simulink model "Controlador_PID_de_movimiento_discreto"  (R2023b)
settings: Solver=VariableStepAuto  StartTime=0.0  StopTime=14  RelTol=1e-3
values from neighbouring files (symbols this model uses):
  alpha_Cu = 3.9e-3    (= 0.0039)    [definicio_cte.m]
  b_a = 0.0396    [definicio_cte.m]
  b_eq = b_m + b_l/(r^2)    (= 1.98611111111e-05)    [definicio_cte.m]
  C_ts = 0.818    [definicio_cte.m]
  g = 9.80665    [definicio_cte.m]
  J_eq = J_m + J_l/(r^2)    (= 1.97847222222e-05)    [definicio_cte.m]
  k_l = m*l_cm + m_l*l_l    (= 0.25)    [definicio_cte.m]
  K_omega_2 = 3.0720e7    (= 30720000)    [definicio_cte.m]
  K_sa = 31.656    [definicio_cte.m]
  K_theta_2 = 9600    [definicio_cte.m]
  K_theta_i = 3.2768e10    (= 32768000000)    [definicio_cte.m]
  L_d = 6.6e-3    (= 0.0066)    [definicio_cte.m]
  L_ls = 0.8e-3    (= 0.0008)    [definicio_cte.m]
  L_q = 5.8e-3    (= 0.0058)    [definicio_cte.m]
  lambda_m = 0.016    [definicio_cte.m]
  lim_inf = -sqrt(2) * 48 / sqrt(3)    [definicio_cte.m]
  lim_sup = sqrt(2) * 48 / sqrt(3)    [definicio_cte.m]
  P_p = 3    [definicio_cte.m]
  r = 120    [definicio_cte.m]
  R_0 = 5000 * L_ls    (= 4)    [definicio_cte.m]
  R_d = 5000 * L_d    (= 33)    [definicio_cte.m]
  R_q = 5000 * L_q    (= 29)    [definicio_cte.m]
  R_sREF = 1.02    [definicio_cte.m]
  R_tsamb = 146.7    [definicio_cte.m]
  T_amb = 25    [definicio_cte.m]
  T_sREF = 20    [definicio_cte.m]
  tau = 20    [definicio_cte.m]
  Ts = 1.256e-4    (= 0.0001256)    [definicio_cte.m]
  w_modul = 6000*4    (= 24000)    [definicio_cte.m]
  wn_i = 6000*3    (= 18000)    [definicio_cte.m]
  wn_theta = 2000*3    (= 6000)    [definicio_cte.m]
  xita_i = 1    [definicio_cte.m]
  xita_modul = 1    [definicio_cte.m]
  xita_theta = 1    [definicio_cte.m]
undefined symbols (not defined in the file or in its folder): K_sia, magnitude
libraries: simulink x16
(part 2 of 2)

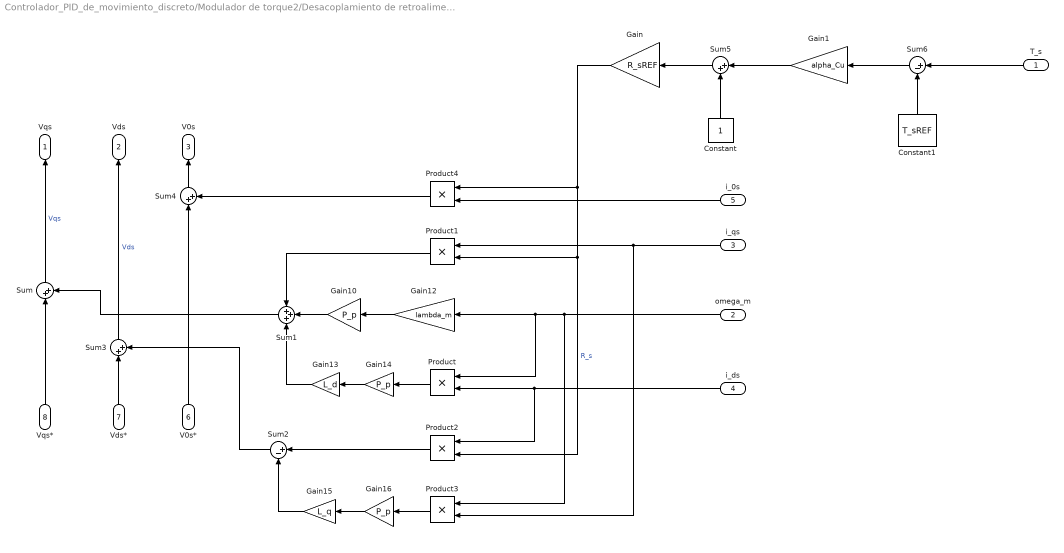
== system Controlador_PID_de_movimiento_discreto/Modulador de torque2/Desacoplamiento de retroalimentaciones fisicas naturales ==
  T_s : Inport
  omega_m : Inport  Port=2
  i_qs : Inport  Port=3
  i_ds : Inport  Port=4
  i_0s : Inport  Port=5
  V0s* : Inport  Port=6
  Vds* : Inport  Port=7
  Vqs* : Inport  Port=8
  Constant : Constant
  Constant1 : Constant  Value=T_sREF
  Gain : Gain  Gain=R_sREF
  Gain1 : Gain  Gain=alpha_Cu
  Gain10 : Gain  Gain=P_p
  Gain12 : Gain  Gain=lambda_m
  Gain13 : Gain  Gain=L_d
  Gain14 : Gain  Gain=P_p
  Gain15 : Gain  Gain=L_q
  Gain16 : Gain  Gain=P_p
  Product{,1..4} (5 alike) : Product
  Sum{,3..5} (4 alike) : Sum  Inputs=|++
  Sum1 : Sum  Inputs=+++
  Sum2 : Sum  Inputs=|+-
  Sum6 : Sum  Inputs=|+-
  Vqs : Outport
  Vds : Outport  Port=2
  V0s : Outport  Port=3
  wires:
  Gain10/1 -> Sum1/2
  Gain13/1 -> Sum1/3
  Gain12/1 -> Gain10/1
  i_qs/1 -> Product3/2, Product1/1
  i_ds/1 -> Product2/1, Product/2
  Gain16/1 -> Gain15/1
  Product2/1 -> Sum2/1
  Product3/1 -> Gain16/1
  Gain/1 -> Product2/2, Product1/2, Product4/1  "R_s"
  Gain15/1 -> Sum2/2
  Product1/1 -> Sum1/1
  Sum2/1 -> Sum3/2
  Sum1/1 -> Sum/2
  Product/1 -> Gain14/1
  omega_m/1 -> Product3/1, Product/1, Gain12/1
  Gain14/1 -> Gain13/1
  Sum3/1 -> Vds/1  "Vds"
  Sum/1 -> Vqs/1  "Vqs"
  i_0s/1 -> Product4/2
  Product4/1 -> Sum4/2
  Sum4/1 -> V0s/1
  Constant1/1 -> Sum6/2
  T_s/1 -> Sum6/1
  Constant/1 -> Sum5/2
  Sum5/1 -> Gain/1
  Sum6/1 -> Gain1/1
  Gain1/1 -> Sum5/1
  Vqs*/1 -> Sum/1
  Vds*/1 -> Sum3/1
  V0s*/1 -> Sum4/1

== system Controlador_PID_de_movimiento_discreto/Modulador de torque2/Lazo de corriente ==
  i_qs : Inport
  i_ds : Inport  Port=2
  i_0s : Inport  Port=3
  iqs* : Inport  Port=4
  ids* : Inport  Port=5
  i0s* : Inport  Port=6
  Gain10 : Gain  Gain=R_d
  Gain12 : Gain  Gain=R_0
  Gain9 : Gain  Gain=R_q
  Sum : Sum  Inputs=|-+
  Sum1 : Sum  Inputs=|-+
  Sum2 : Sum  Inputs=|-+
  V0s* : Outport
  Vds* : Outport  Port=2
  Vqs* : Outport  Port=3
  wires:
  Gain9/1 -> Vqs*/1  "Vqs*"
  Sum/1 -> Gain9/1
  Gain10/1 -> Vds*/1  "Vds*"
  i_qs/1 -> Sum/1
  ids*/1 -> Sum1/2
  i_0s/1 -> Sum2/1
  Sum2/1 -> Gain12/1
  Sum1/1 -> Gain10/1
  i0s*/1 -> Sum2/2
  iqs*/1 -> Sum/2
  i_ds/1 -> Sum1/1
  Gain12/1 -> V0s*/1  "V0s*"

== system Controlador_PID_de_movimiento_discreto/Modulador de torque2/Lazo de torque ==
  omega_m : Inport
  T_m'* : Inport  Port=2
  g : Inport  Port=3
  i_ds : Inport  Port=4
  theta_m : Inport  Port=5
  Constant4 : Constant  Value=L_d
  Constant5 : Constant  Value=L_q
  Constant6 : Constant  Value=lambda_m
  Divide1 : Product  Inputs=*/
  Gain16 : Gain  Gain=b_eq
  Gain17 : Gain  Gain=1/r
  Gain18 : Gain  Gain=k_l
  Gain19 : Gain  Gain=1/r
  Gain20 : Gain  Gain=P_p
  Gain21 : Gain  Gain=3/2
  Product1 : Product
  Product3 : Product
  Sin1 : Trigonometry
  Sum3 : Sum  Inputs=+++
  Sum4 : Sum  Inputs=-+
  Sum5 : Sum  Inputs=|++
  iqs* : Outport
  wires:
  theta_m/1 -> Gain17/1
  Product1/1 -> Sum3/3
  Constant6/1 -> Sum5/2
  Gain16/1 -> Sum3/2
  T_m'*/1 -> Sum3/1
  Gain21/1 -> Divide1/2
  g/1 -> Product1/2
  Constant5/1 -> Sum4/1
  Product3/1 -> Sum5/1
  Sum5/1 -> Gain20/1
  Gain18/1 -> Gain19/1
  Sum3/1 -> Divide1/1
  Divide1/1 -> iqs*/1  "iqs*"
  Gain20/1 -> Gain21/1
  Sum4/1 -> Product3/2
  Gain19/1 -> Product1/1
  Gain17/1 -> Sin1/1
  omega_m/1 -> Gain16/1
  Sin1/1 -> Gain18/1
  i_ds/1 -> Product3/1
  Constant4/1 -> Sum4/2

== system Controlador_PID_de_movimiento_discreto/Subsystem10/Subsystem ==
  u_a : Inport
  Gain10 : Gain  Gain=w_modul
  Gain12 : Gain  Gain=xita_modul
  Gain13 : Gain  Gain=2
  Gain14 : Gain  Gain=(w_modul)^2
  Gain9 : Gain  Gain=(w_modul)^2
  Integrator : Integrator
  Integrator1 : Integrator
  Sum : Sum  Inputs=+--
  y_a : Outport
  wires:
  Integrator1/1 -> y_a/1, Gain14/1  "x_1 = y"
  Integrator/1 -> Gain10/1, Integrator1/1  "x_2 = x_1'"
  Gain12/1 -> Gain13/1
  Gain13/1 -> Sum/3
  Sum/1 -> Integrator/1  "y' = x_2'"
  Gain9/1 -> Sum/1
  Gain10/1 -> Gain12/1
  Gain14/1 -> Sum/2
  u_a/1 -> Gain9/1

== system Controlador_PID_de_movimiento_discreto/Subsystem3/Subsystem ==
  u_a : Inport
  Gain10 : Gain  Gain=w_modul
  Gain12 : Gain  Gain=xita_modul
  Gain13 : Gain  Gain=2
  Gain14 : Gain  Gain=(w_modul)^2
  Gain9 : Gain  Gain=(w_modul)^2
  Integrator : Integrator
  Integrator1 : Integrator
  Sum : Sum  Inputs=+--
  y_a : Outport
  wires:
  Integrator1/1 -> y_a/1, Gain14/1  "x_1 = y"
  Integrator/1 -> Gain10/1, Integrator1/1  "x_2 = x_1'"
  Gain12/1 -> Gain13/1
  Gain13/1 -> Sum/3
  Sum/1 -> Integrator/1  "y' = x_2'"
  Gain9/1 -> Sum/1
  Gain10/1 -> Gain12/1
  Gain14/1 -> Sum/2
  u_a/1 -> Gain9/1

== system Controlador_PID_de_movimiento_discreto/Subsystem4/Subsystem ==
  u_a : Inport
  Gain10 : Gain  Gain=w_modul
  Gain12 : Gain  Gain=xita_modul
  Gain13 : Gain  Gain=2
  Gain14 : Gain  Gain=(w_modul)^2
  Gain9 : Gain  Gain=(w_modul)^2
  Integrator : Integrator
  Integrator1 : Integrator
  Sum : Sum  Inputs=+--
  y_a : Outport
  wires:
  u_a/1 -> Gain9/1
  Gain14/1 -> Sum/2
  Gain10/1 -> Gain12/1
  Gain9/1 -> Sum/1
  Sum/1 -> Integrator/1  "y' = x_2'"
  Gain13/1 -> Sum/3
  Gain12/1 -> Gain13/1
  Integrator/1 -> Integrator1/1, Gain10/1  "x_2 = x_1'"
  Integrator1/1 -> Gain14/1, y_a/1  "x_1 = y"

== system Controlador_PID_de_movimiento_discreto/Subsystem5/Subsystem ==
  u_a : Inport
  Gain10 : Gain  Gain=w_modul
  Gain12 : Gain  Gain=xita_modul
  Gain13 : Gain  Gain=2
  Gain14 : Gain  Gain=(w_modul)^2
  Gain9 : Gain  Gain=(w_modul)^2
  Integrator : Integrator
  Integrator1 : Integrator
  Sum : Sum  Inputs=+--
  y_a : Outport
  wires:
  Integrator1/1 -> y_a/1, Gain14/1  "x_1 = y"
  Integrator/1 -> Gain10/1, Integrator1/1  "x_2 = x_1'"
  Gain12/1 -> Gain13/1
  Gain13/1 -> Sum/3
  Sum/1 -> Integrator/1  "y' = x_2'"
  Gain9/1 -> Sum/1
  Gain10/1 -> Gain12/1
  Gain14/1 -> Sum/2
  u_a/1 -> Gain9/1

== system Controlador_PID_de_movimiento_discreto/Subsystem8/Subsystem ==
  u_a : Inport
  Gain10 : Gain  Gain=w_modul
  Gain12 : Gain  Gain=xita_modul
  Gain13 : Gain  Gain=2
  Gain14 : Gain  Gain=(w_modul)^2
  Gain9 : Gain  Gain=(w_modul)^2
  Integrator : Integrator
  Integrator1 : Integrator
  Sum : Sum  Inputs=+--
  y_a : Outport
  wires:
  Integrator1/1 -> y_a/1, Gain14/1  "x_1 = y"
  Integrator/1 -> Gain10/1, Integrator1/1  "x_2 = x_1'"
  Gain12/1 -> Gain13/1
  Gain13/1 -> Sum/3
  Sum/1 -> Integrator/1  "y' = x_2'"
  Gain9/1 -> Sum/1
  Gain10/1 -> Gain12/1
  Gain14/1 -> Sum/2
  u_a/1 -> Gain9/1

== system Controlador_PID_de_movimiento_discreto/Subsystem9/Subsystem ==
  u_a : Inport
  Gain10 : Gain  Gain=w_modul
  Gain12 : Gain  Gain=xita_modul
  Gain13 : Gain  Gain=2
  Gain14 : Gain  Gain=(w_modul)^2
  Gain9 : Gain  Gain=(w_modul)^2
  Integrator : Integrator
  Integrator1 : Integrator
  Sum : Sum  Inputs=+--
  y_a : Outport
  wires:
  u_a/1 -> Gain9/1
  Gain14/1 -> Sum/2
  Gain10/1 -> Gain12/1
  Gain9/1 -> Sum/1
  Sum/1 -> Integrator/1  "y' = x_2'"
  Gain13/1 -> Sum/3
  Gain12/1 -> Gain13/1
  Integrator/1 -> Integrator1/1, Gain10/1  "x_2 = x_1'"
  Integrator1/1 -> Gain14/1, y_a/1  "x_1 = y"

== system Controlador_PID_de_movimiento_discreto/observador de estados 1/Integrador discreto ==
  u : Inport
  Gain : Gain  Gain=Ts/2
  Sum : Sum  Inputs=|++
  Sum1 : Sum  Inputs=|++
  Unit Delay : UnitDelay  SampleTime=Ts  HasFrameUpgradeWarning=on
  Unit Delay1 : UnitDelay  SampleTime=Ts  HasFrameUpgradeWarning=on
  y : Outport
  wires:
  Unit Delay/1 -> Sum1/2
  Gain/1 -> Sum1/1
  Unit Delay1/1 -> Sum/2
  u/1 -> Unit Delay1/1, Sum/1
  Sum1/1 -> y/1, Unit Delay/1
  Sum/1 -> Gain/1

== system Controlador_PID_de_movimiento_discreto/observador de estados 1/Integrador discreto1 ==
  u : Inport
  Gain : Gain  Gain=Ts/2
  Sum : Sum  Inputs=|++
  Sum1 : Sum  Inputs=|++
  Unit Delay : UnitDelay  SampleTime=Ts  HasFrameUpgradeWarning=on
  Unit Delay1 : UnitDelay  SampleTime=Ts  HasFrameUpgradeWarning=on
  y : Outport
  wires:
  Sum/1 -> Gain/1
  Sum1/1 -> Unit Delay/1, y/1
  u/1 -> Sum/1, Unit Delay1/1
  Unit Delay1/1 -> Sum/2
  Gain/1 -> Sum1/1
  Unit Delay/1 -> Sum1/2

== system Controlador_PID_de_movimiento_discreto/observador de estados 1/Integrador discreto2 ==
  u : Inport
  Gain : Gain  Gain=Ts/2
  Sum : Sum  Inputs=|++
  Sum1 : Sum  Inputs=|++
  Unit Delay : UnitDelay  SampleTime=Ts  HasFrameUpgradeWarning=on
  Unit Delay1 : UnitDelay  SampleTime=Ts  HasFrameUpgradeWarning=on
  y : Outport
  wires:
  Unit Delay/1 -> Sum1/2
  Gain/1 -> Sum1/1
  Unit Delay1/1 -> Sum/2
  u/1 -> Unit Delay1/1, Sum/1
  Sum1/1 -> y/1, Unit Delay/1
  Sum/1 -> Gain/1

== system Controlador_PID_de_movimiento_discreto/./Subsistema Electromagnético/corriente_i_0s ==
  v_0s : Inport
  R_s : Inport  Port=2
  Gain : Gain  Gain=1/L_ls
  Integrator : Integrator
  Product : Product
  Sum : Sum  Inputs=+-
  i_0s : Outport
  wires:
  Sum/1 -> Gain/1
  Gain/1 -> Integrator/1  "i'_0s"
  Integrator/1 -> i_0s/1, Product/2
  Product/1 -> Sum/2
  v_0s/1 -> Sum/1
  R_s/1 -> Product/1

== system Controlador_PID_de_movimiento_discreto/./Subsistema Electromagnético/corriente_i_ds ==
  v_ds : Inport
  i_qs : Inport  Port=2
  omega_m : Inport  Port=3
  R_s : Inport  Port=4
  Gain : Gain  Gain=L_q
  Gain1 : Gain  Gain=P_p
  Gain2 : Gain  Gain=1/L_d
  Integrator1 : Integrator
  Product : Product
  Product2 : Product
  Sum : Sum  Inputs=++-
  i_ds : Outport
  wires:
  Gain1/1 -> Product/2
  Gain/1 -> Product/1
  i_qs/1 -> Gain/1
  Product/1 -> Sum/2
  Integrator1/1 -> i_ds/1, Product2/2
  v_ds/1 -> Sum/1
  Gain2/1 -> Integrator1/1  "i'_ds"
  R_s/1 -> Product2/1
  Sum/1 -> Gain2/1
  Product2/1 -> Sum/3
  omega_m/1 -> Gain1/1

== system Controlador_PID_de_movimiento_discreto/./Subsistema Electromagnético/corriente_i_qs ==
  omega_m : Inport
  v_qs : Inport  Port=2
  R_s : Inport  Port=3
  i_ds : Inport  Port=4
  Constant : Constant  Value=lambda_m
  Gain : Gain  Gain=P_p
  Gain1 : Gain  Gain=L_d
  Gain2 : Gain  Gain=1/L_q
  Integrator1 : Integrator
  Product : Product
  Product1 : Product
  Sum : Sum  Inputs=+--
  Sum1 : Sum  Inputs=++|
  i_qs : Outport
  wires:
  Gain1/1 -> Sum1/2
  Product/1 -> Sum/2
  R_s/1 -> Product/2
  Sum1/1 -> Product1/1
  v_qs/1 -> Sum/1
  Gain/1 -> Product1/2
  Gain2/1 -> Integrator1/1  "i'qs"
  Constant/1 -> Sum1/1
  i_ds/1 -> Gain1/1
  Sum/1 -> Gain2/1
  omega_m/1 -> Gain/1
  Integrator1/1 -> i_qs/1, Product/1
  Product1/1 -> Sum/3

== system Controlador_PID_de_movimiento_discreto/./Subsistema Electromagnético/torque_T_m ==
  i_ds : Inport
  i_qs : Inport  Port=2
  Constant : Constant  Value=lambda_m
  Gain : Gain  Gain=L_d-L_q
  Gain1 : Gain  Gain=3/2
  Gain2 : Gain  Gain=P_p
  Product : Product
  Sum : Sum  Inputs=++|
  T_m : Outport
  wires:
  Constant/1 -> Sum/1
  Gain/1 -> Sum/2
  i_ds/1 -> Gain/1
  Product/1 -> Gain1/1
  i_qs/1 -> Product/2
  Sum/1 -> Product/1
  Gain1/1 -> Gain2/1
  Gain2/1 -> T_m/1

== system Controlador_PID_de_movimiento_discreto/.1/Subsistema Electromagnético/corriente_i_0s ==
  v_0s : Inport
  R_s : Inport  Port=2
  Gain : Gain  Gain=1/L_ls
  Integrator : Integrator
  Product : Product
  Sum : Sum  Inputs=+-
  i_0s : Outport
  wires:
  Sum/1 -> Gain/1
  Gain/1 -> Integrator/1  "i'_0s"
  Integrator/1 -> i_0s/1, Product/2
  Product/1 -> Sum/2
  v_0s/1 -> Sum/1
  R_s/1 -> Product/1

== system Controlador_PID_de_movimiento_discreto/.1/Subsistema Electromagnético/corriente_i_ds ==
  v_ds : Inport
  i_qs : Inport  Port=2
  omega_m : Inport  Port=3
  R_s : Inport  Port=4
  Gain : Gain  Gain=L_q
  Gain1 : Gain  Gain=P_p
  Gain2 : Gain  Gain=1/L_d
  Integrator1 : Integrator
  Product : Product
  Product2 : Product
  Sum : Sum  Inputs=++-
  i_ds : Outport
  wires:
  Gain1/1 -> Product/2
  Gain/1 -> Product/1
  i_qs/1 -> Gain/1
  Product/1 -> Sum/2
  Integrator1/1 -> i_ds/1, Product2/2
  v_ds/1 -> Sum/1
  Gain2/1 -> Integrator1/1  "i'_ds"
  R_s/1 -> Product2/1
  Sum/1 -> Gain2/1
  Product2/1 -> Sum/3
  omega_m/1 -> Gain1/1

== system Controlador_PID_de_movimiento_discreto/.1/Subsistema Electromagnético/corriente_i_qs ==
  omega_m : Inport
  v_qs : Inport  Port=2
  R_s : Inport  Port=3
  i_ds : Inport  Port=4
  Constant : Constant  Value=lambda_m
  Gain : Gain  Gain=P_p
  Gain1 : Gain  Gain=L_d
  Gain2 : Gain  Gain=1/L_q
  Integrator1 : Integrator
  Product : Product
  Product1 : Product
  Sum : Sum  Inputs=+--
  Sum1 : Sum  Inputs=++|
  i_qs : Outport
  wires:
  Gain1/1 -> Sum1/2
  Product/1 -> Sum/2
  R_s/1 -> Product/2
  Sum1/1 -> Product1/1
  v_qs/1 -> Sum/1
  Gain/1 -> Product1/2
  Gain2/1 -> Integrator1/1  "i'qs"
  Constant/1 -> Sum1/1
  i_ds/1 -> Gain1/1
  Sum/1 -> Gain2/1
  omega_m/1 -> Gain/1
  Integrator1/1 -> i_qs/1, Product/1
  Product1/1 -> Sum/3

== system Controlador_PID_de_movimiento_discreto/.1/Subsistema Electromagnético/torque_T_m ==
  i_ds : Inport
  i_qs : Inport  Port=2
  Constant : Constant  Value=lambda_m
  Gain : Gain  Gain=L_d-L_q
  Gain1 : Gain  Gain=3/2
  Gain2 : Gain  Gain=P_p
  Product : Product
  Sum : Sum  Inputs=++|
  T_m : Outport
  wires:
  Constant/1 -> Sum/1
  Gain/1 -> Sum/2
  i_ds/1 -> Gain/1
  Product/1 -> Gain1/1
  i_qs/1 -> Product/2
  Sum/1 -> Product/1
  Gain1/1 -> Gain2/1
  Gain2/1 -> T_m/1

== matlab function Controlador_PID_de_movimiento_discreto/MATLAB Function2 ==
  data: f_qs input; f_as output; theta_r input; f_ds input; f_0s input; f_bs output; f_cs output
function [f_as, f_bs, f_cs] = inversa_park(f_qs, theta_r, f_ds, f_0s)
    % =====================================================================
    % TRANSFORMACION INVERSA DE PARK
    % Descripción: Convierte variables del marco de referencia síncrono (q, d, 0)
    %              al marco de referencia estacionario trifásico (a, b, c).
    % =====================================================================

    % 1. VARIABLES PARA PRECÁLCULO
    persistent DOS_PI_TERCIOS;

    % 2. INICIALIZACIÓN Y PRECÁLCULO (Instante k=0)
    if isempty(DOS_PI_TERCIOS)
        % Calculamos el desfase de 120° en radianes una sola vez
        DOS_PI_TERCIOS = (2 * pi) / 3;
    end

    % 3. CÁLCULO DE LOS ÁNGULOS DESFASADOS
    theta_a = theta_r;
    theta_b = theta_r - DOS_PI_TERCIOS;
    theta_c = theta_r + DOS_PI_TERCIOS;

    % 4. LEY DE TRANSFORMACIÓN (Funciones escalares desagregadas)
    
    % --- Fase A ---
    comp_q_a = f_qs * cos(theta_a);
    comp_d_a = f_ds * sin(theta_a);
    f_as = comp_q_a + comp_d_a + f_0s;

    % --- Fase B ---
    comp_q_b = f_qs * cos(theta_b);
    comp_d_b = f_ds * sin(theta_b);
    f_bs = comp_q_b + comp_d_b + f_0s;

    % --- Fase C ---
    comp_q_c = f_qs * cos(theta_c);
    comp_d_c = f_ds * sin(theta_c);
    f_cs = comp_q_c + comp_d_c + f_0s;

end

== matlab function Controlador_PID_de_movimiento_discreto/MATLAB Function3 ==
  data: f_as input; f_qs output; f_bs input; f_cs input; theta_r input; f_ds output; f_0s output
function [f_qs, f_ds, f_0s] = directa_park(f_as, f_bs, f_cs, theta_r)
    % =====================================================================
    % TRANSFORMACION DIRECTA DE PARK
    % Descripción: Convierte variables del marco estacionario trifásico 
    %              (a, b, c) al marco de referencia síncrono (q, d, 0).
    % =====================================================================

    % 1. VARIABLES PARA PRECÁLCULO
    persistent DOS_PI_TERCIOS DOS_TERCIOS UN_TERCIO;

    % 2. INICIALIZACIÓN Y PRECÁLCULO (Instante k=0)
    if isempty(DOS_PI_TERCIOS)
        % Calculamos constantes y divisiones una sola vez
        DOS_PI_TERCIOS = (2 * pi) / 3;
        DOS_TERCIOS = 2 / 3;
        UN_TERCIO = 1 / 3;
    end

    % 3. CÁLCULO DE LOS ÁNGULOS DESFASADOS
    theta_a = theta_r;
    theta_b = theta_r - DOS_PI_TERCIOS;
    theta_c = theta_r + DOS_PI_TERCIOS;

    % 4. LEY DE TRANSFORMACIÓN (Funciones escalares desagregadas)
    
    % --- Eje q ---
    comp_q_a = f_as * cos(theta_a);
    comp_q_b = f_bs * cos(theta_b);
    comp_q_c = f_cs * cos(theta_c);
    f_qs = DOS_TERCIOS * (comp_q_a + comp_q_b + comp_q_c);

    % --- Eje d ---
    comp_d_a = f_as * sin(theta_a);
    comp_d_b = f_bs * sin(theta_b);
    comp_d_c = f_cs * sin(theta_c);
    f_ds = DOS_TERCIOS * (comp_d_a + comp_d_b + comp_d_c);

    % --- Eje 0 (Secuencia Cero) ---
    suma_abc = f_as + f_bs + f_cs;
    f_0s = UN_TERCIO * suma_abc;

end

== matlab function Controlador_PID_de_movimiento_discreto/MATLAB Function1 ==
  data: T_m_ref input; omega_obs output; theta_m input; theta_obs output; Ts parameter; J_eq parameter; K_theta_i parameter; K_omega_2 parameter; K_theta_2 parameter
function [omega_obs, theta_obs] = observador_estados(T_m_ref, theta_m, Ts, J_eq, K_theta_i, K_omega_2, K_theta_2)
    % =====================================================================
    % OBSERVADOR DE ESTADOS DISCRETO
    % Descripción: Estima velocidad (omega_obs) y posición (theta_obs) 
    %              usando integración trapezoidal (Tustin).
    % Entradas:
    %   T_m_ref    : Torque de referencia (del controlador anterior)
    %   theta_m    : Posición medida
    % Parámetros (Scope -> Parameter en Simulink):
    %   Ts, J_eq, K_theta_i, K_omega_2, K_theta_2
    % Salidas:
    %   omega_obs  : Velocidad estimada
    %   theta_obs  : Posición estimada
    % =====================================================================

    % 1. DECLARACIÓN DE ESTADOS INTERNOS (Memoria estática)
    
    % Integrador 1 (Rama izquierda: Perturbación 'v')
    % Entrada: dv | Salida: v
    persistent dv_anterior v_anterior;
    
    % Integrador 2 (Rama central: Aceleración -> Velocidad)
    % Entrada: domega_obs | Salida: omega_obs
    persistent domega_obs_anterior omega_obs_anterior;
    
    % Integrador 3 (Rama derecha: Velocidad -> Posición)
    % Entrada: dtheta_obs | Salida: theta_obs
    persistent dtheta_obs_anterior theta_obs_anterior;
    
    % Constantes precálculadas
    persistent K_tustin inv_J_eq;

    % 2. INICIALIZACIÓN Y PRECÁLCULO (Instante k=0)
    if isempty(dv_anterior)
        % Inicialización de estados a cero
        dv_anterior = 0; 
        v_anterior = 0;
        
        domega_obs_anterior = 0; 
        omega_obs_anterior = 0;
        
        dtheta_obs_anterior = 0; 
        theta_obs_anterior = 0;
        
        % PRECÁLCULOS: 
        K_tustin = Ts / 2;
        inv_J_eq = 1 / J_eq; % Transformamos la división en una multiplicación
    end

    % 3. CÁLCULO DE LA LEY DEL OBSERVADOR (Secuencial)
    
    % a. Cálculo del error de estimación
    % Usamos theta_obs_anterior (la estimación del ciclo pasado) 
    % para evaluar el error actual y evitar bucles algebraicos.
    e_obs_theta = theta_m - theta_obs_anterior;
    
    % b. Rama 1: Integrador de perturbación (izquierda)
    dv = e_obs_theta * K_theta_i;
    suma_dv = dv + dv_anterior;
    v = v_anterior + (K_tustin * suma_dv);
    
    % c. Rama 2: Estimador de Velocidad (centro)
    % Sumatoria de nodos antes del integrador 1
    aceleracion_ref = T_m_ref * inv_J_eq;
    domega_obs = aceleracion_ref + v + (e_obs_theta * K_omega_2);
    
    % Tustin Integrador 1
    suma_domega = domega_obs + domega_obs_anterior;
    omega_obs = omega_obs_anterior + (K_tustin * suma_domega);
    
    % d. Rama 3: Estimador de Posición (derecha)
    % Sumatoria de nodos antes del integrador 2
    dtheta_obs = omega_obs + (e_obs_theta * K_theta_2);
    
    % Tustin Integrador 2
    suma_dtheta = dtheta_obs + dtheta_obs_anterior;
    theta_obs = theta_obs_anterior + (K_tustin * suma_dtheta);

    % 4. ACTUALIZACIÓN DE ESTADOS (Para el ciclo k+1)
    dv_anterior = dv;
    v_anterior = v;
    
    domega_obs_anterior = domega_obs;
    omega_obs_anterior = omega_obs;
    
    dtheta_obs_anterior = dtheta_obs;
    theta_obs_anterior = theta_obs;
    
end

== matlab function Controlador_PID_de_movimiento_discreto/MATLAB Function ==
  data: omega_m input; T_m_ref output; omega_m_ref input; Ts parameter; K_sia parameter; K_sa parameter; b_a parameter
function T_m_ref = controlador_pid_movimiento(omega_m, omega_m_ref, Ts, K_sia, K_sa, b_a)
    % =====================================================================
    % CONTROLADOR PID DE MOVIMIENTO DISCRETO
    % Descripción: Controlador de posición/velocidad con doble integrador
    %              por método trapezoidal (Tustin).
    % =====================================================================

    % 1. DECLARACIÓN DE ESTADOS INTERNOS (Memoria estática)
    
    % Memoria del Integrador 1 (Velocidad -> Posición)
    persistent e_omega_m_anterior;
    
    % Memoria compartida: Es la salida del Int 1 y la entrada del Int 2
    persistent e_theta_anterior;
    
    % Memoria del Integrador 2 (Posición -> Integral de Posición)
    persistent integral_e_theta_anterior;
    
    % Constante precálculada
    persistent K_tustin;

    % 2. INICIALIZACIÓN Y PRECÁLCULO (Se ejecuta solo en el instante k=0)
    if isempty(e_omega_m_anterior)
        % Inicializar memorias a cero (reposo)
        e_omega_m_anterior = 0;
        e_theta_anterior = 0;
        integral_e_theta_anterior = 0;
        
        % PRECÁLCULO: Se resuelve la constante una sola vez
        K_tustin = Ts / 2;
    end

    % 3. CÁLCULO DE LA LEY DE CONTROL (Funciones escalares)
    
    % a. Error de velocidad actual
    e_omega_m = omega_m_ref - omega_m;
    
    % b. Acción derivativa/velocidad (rama inferior)
    accion_v = e_omega_m * b_a;
    
    % c. Integrador 1: Cálculo del error de posición actual (e_theta)
    suma_e_omega_m = e_omega_m + e_omega_m_anterior;
    delta_area_int1 = K_tustin * suma_e_omega_m;
    e_theta = e_theta_anterior + delta_area_int1;
    
    % d. Acción proporcional/posición (rama central)
    accion_p = e_theta * K_sa;
    
    % e. Integrador 2: Cálculo de la integral de posición actual
    % Nota como reciclamos "e_theta_anterior" porque es la misma señal
    suma_e_theta = e_theta + e_theta_anterior;
    delta_area_int2 = K_tustin * suma_e_theta;
    integral_e_theta = integral_e_theta_anterior + delta_area_int2;
    
    % f. Acción integral/posición (rama superior)
    accion_i = integral_e_theta * K_sia;
    
    % g. Suma final (Torque de referencia)
    T_m_ref = accion_i + accion_p + accion_v;

    % 4. ACTUALIZACIÓN DE ESTADOS (Para el ciclo k+1)
    e_omega_m_anterior = e_omega_m;
    e_theta_anterior = e_theta;
    integral_e_theta_anterior = integral_e_theta;
    
end

== matlab function Controlador_PID_de_movimiento_discreto/Modulador de torque/MATLAB Function2 ==
  data: omega_obs input; iqs_ref output; theta_m input; T_m_ref input; g input; i_ds input; k_l parameter; L_d parameter; L_q parameter; P_p parameter; lambda_m parameter; r parameter; b_eq parameter
function iqs_ref = lazo_de_torque(omega_obs, theta_m, T_m_ref, g, i_ds, k_l, L_d, L_q, P_p, lambda_m, r, b_eq)
    % =====================================================================
    % LAZO DE TORQUE DISCRETO (Optimizado)
    % Se eliminó el integrador interno. Recibe posición (theta_m) y 
    % velocidad (omega_obs) directamente de los bloques anteriores.
    % =====================================================================

    % Variables para el precálculo de constantes
    persistent inv_r K_seno L_diff K_denominador;

    % INICIALIZACIÓN Y PRECÁLCULO (Instante k=0)
    if isempty(inv_r)
        % PRECÁLCULOS: Agrupamos todas las constantes posibles
        inv_r = 1 / r;                 % Para el argumento del seno
        K_seno = k_l / r;              % Ganancia combinada fuera del seno
        L_diff = L_d - L_q;            % Resta de inductancias
        K_denominador = 1.5 * P_p;     % Ganancias de la rama inferior (3/2 * P_p)
    end

    % 1. Cálculo del Numerador (Suma de las 3 ramas superiores)
    % Rama 1: T_m_ref (Torque de referencia)
    
    % Rama 2: Fricción equivalente (usando la velocidad estimada)
    termino_b = omega_obs * b_eq;
    
    % Rama 3: Efecto de la gravedad (usando la posición medida pura)
    argumento_seno = theta_m * inv_r;
    termino_g = g * K_seno * sin(argumento_seno);
    
    numerador = T_m_ref + termino_b + termino_g;
    
    % 2. Cálculo del Denominador (Rama inferior)
    parentesis_den = (L_diff * i_ds) + lambda_m;
    denominador = K_denominador * parentesis_den;
    
    % 3. Salida final
    iqs_ref = numerador / denominador;
    
end

== matlab function Controlador_PID_de_movimiento_discreto/Modulador de torque/MATLAB Function3 ==
  data: i_qs input; V0s_ref output; i_ds input; i_0s input; iqs_ref input; ids_ref input; i0s_ref input; Vds_ref output; Vqs_ref output; R_q parameter; R_d parameter; R_0 parameter
function [V0s_ref, Vds_ref, Vqs_ref] = lazo_de_corriente(i_qs, i_ds, i_0s, iqs_ref, ids_ref, i0s_ref, R_q, R_d, R_0)
    % =====================================================================
    % LAZO DE CORRIENTE DISCRETO
    % Descripción: Controladores puramente proporcionales para las 
    %              corrientes en los ejes d, q y 0.
    % =====================================================================

    % 1. CÁLCULO DE ERRORES
    % Se compara la referencia (setpoint) con la medición actual
    e_i0s = i0s_ref - i_0s;
    e_ids = ids_ref - i_ds;
    e_iqs = iqs_ref - i_qs;

    % 2. LEY DE CONTROL (Acción Proporcional)
    % Se multiplica el error por la ganancia correspondiente a cada eje
    V0s_ref = e_i0s * R_0;
    Vds_ref = e_ids * R_d;
    Vqs_ref = e_iqs * R_q;

end

== matlab function Controlador_PID_de_movimiento_discreto/Modulador de torque/MATLAB Function4 ==
  data: T_stator input; V0s output; omega_m input; i_qs input; i_ds input; i_0s input; V0s_ref input; Vds_ref input; Vqs_ref input; Vds output; Vqs output; R_sREF parameter; alpha_Cu parameter; P_p parameter; L_d parameter; lambda_m parameter; L_q parameter; T_sREF parameter
function [V0s, Vds, Vqs] = desacoplo_retroalimentaciones(T_stator, omega_m, i_qs, i_ds, i_0s, V0s_ref, Vds_ref, Vqs_ref, R_sREF, alpha_Cu, P_p, L_d, lambda_m, L_q, T_sREF)
    % =====================================================================
    % DESACOPLAMIENTO DE RETROALIMENTACIONES FÍSICAS NATURALES
    % Descripción: Compensa la fuerza contraelectromotriz (BEMF), el 
    %              acoplamiento cruzado de los ejes d-q, y la variación de 
    %              la resistencia estatórica por temperatura.
    % =====================================================================

    % 1. VARIABLES PARA PRECÁLCULO
    % Solo guardamos combinaciones de constantes del motor
    persistent K_Ld K_Lq K_lambda;

    % 2. INICIALIZACIÓN Y PRECÁLCULO (Instante k=0)
    if isempty(K_Ld)
        % Multiplicamos las inductancias y el flujo por el número de pares de polos
        K_Ld = L_d * P_p;
        K_Lq = L_q * P_p;
        K_lambda = lambda_m * P_p;
    end

    % 3. CÁLCULO DE LA RESISTENCIA DEPENDIENTE DE LA TEMPERATURA
    % R_s = R_sREF * (1 + alpha_Cu * (T_stator - T_sREF))
    delta_T = T_stator - T_sREF;
    R_s = R_sREF * (1 + (alpha_Cu * delta_T));

    % 4. CÁLCULO DE LAS TENSIONES DESACOPLADAS (Funciones escalares)
    
    % --- Eje 0 ---
    % Caída de tensión resistiva pura
    comp_0s = R_s * i_0s;
    V0s = V0s_ref + comp_0s;

    % --- Eje d ---
    % Caída resistiva - Acoplamiento cruzado del eje q
    % Nota: El diagrama muestra que el término cruzado de L_q se resta
    comp_ds = (R_s * i_ds) - (K_Lq * omega_m * i_qs);
    Vds = Vds_ref + comp_ds;

    % --- Eje q ---
    % Caída resistiva + Acoplamiento cruzado del eje d + Fuerza contraelectromotriz
    comp_qs = (R_s * i_qs) + (K_Ld * omega_m * i_ds) + (K_lambda * omega_m);
    Vqs = Vqs_ref + comp_qs;

end
